simulink model "test_limit_rate"  (Simulink 7.6)
settings: Solver=ode45  StartTime=0.0  StopTime=1000.0  RelTol=1e-3
libraries: simulink x8
settings Model: Creator=jporter  LastModifiedBy=jporter

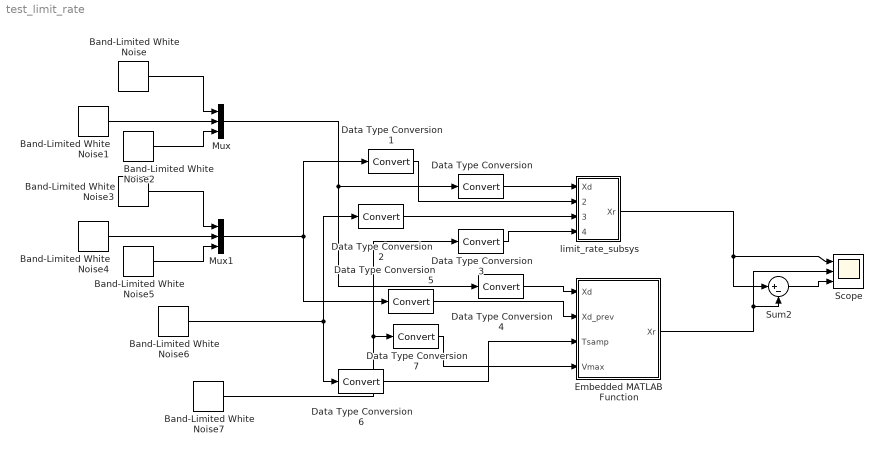
== system test_limit_rate ==
  Band-Limited White Noise{,1..5} (6 alike) : simulink/Sources/Band-Limited White Noise  SystemSampleTime=-1  Cov=0.5  Ts=0.01  seed=[23341]
  Band-Limited White Noise6 : simulink/Sources/Band-Limited White Noise  SystemSampleTime=-1  Cov=0.5  Ts=7  seed=[23341]
  Band-Limited White Noise7 : simulink/Sources/Band-Limited White Noise  SystemSampleTime=-1  Cov=0.5  Ts=10  seed=[23341]
  Data Type Conversion{,1..7} (8 alike) : DataTypeConversion
  Embedded MATLAB Function : Stateflow chart  TreatAsAtomicUnit=on
  Mux : Mux  Inputs=3
  Mux1 : Mux  Inputs=3
  Scope : Scope  NumInputPorts=3
      settings: YMin=-5~-5~-5  YMax=5~5~5
  Sum2 : Sum  Inputs=|+-
  limit_rate_subsys : Subsystem
  wires:
  Mux/1 -> Data Type Conversion/1, Data Type Conversion4/1
  Mux1/1 -> Data Type Conversion1/1, Data Type Conversion5/1
  Band-Limited White Noise6/1 -> Data Type Conversion2/1, Data Type Conversion6/1
  Band-Limited White Noise7/1 -> Data Type Conversion3/1, Data Type Conversion7/1
  Data Type Conversion/1 -> limit_rate_subsys/1(Xd)
  Data Type Conversion1/1 -> limit_rate_subsys/2(Xd_prev)
  Data Type Conversion2/1 -> limit_rate_subsys/3(Tsamp)
  Data Type Conversion3/1 -> limit_rate_subsys/4(Vmax)
  Data Type Conversion4/1 -> Embedded MATLAB Function/1(Xd)
  Data Type Conversion5/1 -> Embedded MATLAB Function/2(Xd_prev)
  Data Type Conversion6/1 -> Embedded MATLAB Function/3(Tsamp)
  Data Type Conversion7/1 -> Embedded MATLAB Function/4(Vmax)
  limit_rate_subsys/1(Xr) -> Scope/1, Sum2/1
  Sum2/1 -> Scope/3
  Embedded MATLAB Function/1(Xr) -> Scope/2, Sum2/2
  Band-Limited White Noise/1 -> Mux/1
  Band-Limited White Noise1/1 -> Mux/2
  Band-Limited White Noise2/1 -> Mux/3
  Band-Limited White Noise3/1 -> Mux1/1
  Band-Limited White Noise4/1 -> Mux1/2
  Band-Limited White Noise5/1 -> Mux1/3

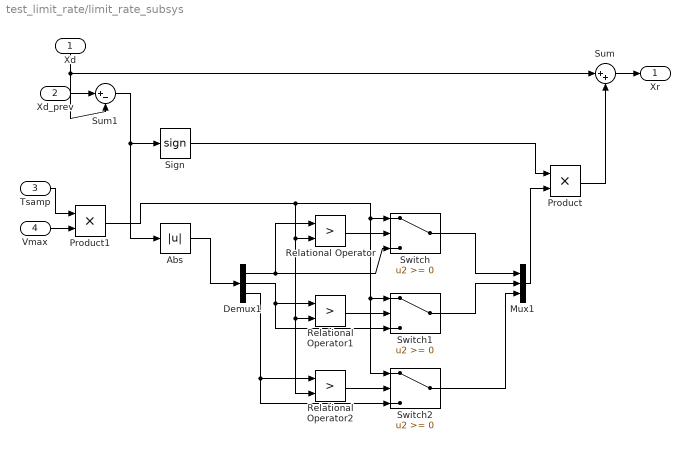
== system test_limit_rate/limit_rate_subsys ==
  Xd : Inport
  Xd_prev : Inport  Port=2
  Tsamp : Inport  Port=3
  Vmax : Inport  Port=4
  Abs : Abs
  Demux1 : Demux  Outputs=3
  Mux1 : Mux  Inputs=3
  Product : Product  RndMeth=Zero
  Product1 : Product  RndMeth=Zero
  Relational Operator : RelationalOperator  Operator=>  OutDataTypeStr=boolean
  Relational Operator1 : RelationalOperator  Operator=>  OutDataTypeStr=boolean
  Relational Operator2 : RelationalOperator  Operator=>  OutDataTypeStr=boolean
  Sign : Signum
  Sum : Sum  Inputs=|++
  Sum1 : Sum  Inputs=|+-
  Switch : Switch
  Switch1 : Switch
  Switch2 : Switch
  Xr : Outport
  wires:
  Xd/1 -> Sum1/2, Sum/1
  Sum1/1 -> Sign/1, Abs/1
  Sign/1 -> Product/1
  Relational Operator/1 -> Switch/2
  Demux1/1 -> Switch/3, Relational Operator/1
  Switch/1 -> Mux1/1
  Abs/1 -> Demux1/1
  Product1/1 -> Relational Operator/2, Relational Operator1/2, Relational Operator2/2, Switch/1, Switch1/1, Switch2/1
  Relational Operator1/1 -> Switch1/2
  Demux1/2 -> Relational Operator1/1, Switch1/3
  Switch1/1 -> Mux1/2
  Relational Operator2/1 -> Switch2/2
  Demux1/3 -> Relational Operator2/1, Switch2/3
  Switch2/1 -> Mux1/3
  Mux1/1 -> Product/2
  Product/1 -> Sum/2
  Sum/1 -> Xr/1
  Xd_prev/1 -> Sum1/1
  Tsamp/1 -> Product1/1
  Vmax/1 -> Product1/2

== matlab function Embedded MATLAB Function ==
  data: Xd input single size=[3]; Xr output single; Xd_prev input single size=[3]; Tsamp input single size=[1]; Vmax input single size=[1]
function Xr = limit_rate(Xd, Xd_prev, Tsamp, Vmax)
% This block supports the Embedded MATLAB subset.
% See the help menu for details. 

delta = Xd - Xd_prev;
delta = sign(delta) .* min( abs(delta), (ones(3,1) * Tsamp * Vmax) );

Xr = Xd_prev + delta;
